simulink model "FitzHugh_Nagumo"  (R2014b)
settings: Solver=ode45  StartTime=0.0  StopTime=100.0  RelTol=1e-3
values from neighbouring files (symbols this model uses):
  a = 0.95    [Run_Aizawa.m]    (also in Run_Arneodo.m = -5.5; Run_Chen.m = 33; Run_Chua.m = 15.6; Run_Chua_4D.m = 0.03)
  A = 30    [Run_Chua_4D.m]    (also in Run_FitzHugh_Nagumo.m = 0.8)
  b = 0.7    [Run_Aizawa.m]    (also in Run_Arneodo.m = 3.5; Run_Chen.m = 3; Run_Chua.m = 28; Run_Duffing.m = 100)
  e = 0.15    [Run_Aizawa.m]    (also in Run_Belousov_Zhabotinsky.m = 0.3; Run_Dadras.m = 9; Run_FitzHugh_Nagumo.m = 0.1)
  omega = 0.7    [Run_FitzHugh_Nagumo.m]
undefined symbols (not defined in the file or in its folder): param
settings Model: Creator=Arek  LastModifiedBy=Arek

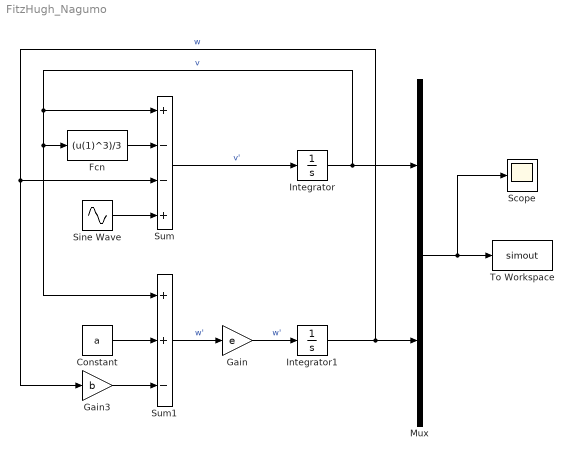
== system FitzHugh_Nagumo ==
  Constant : Constant  Value=a
  Fcn : Fcn  Expr=(u(1)^3)/3
  Gain : Gain  Gain=e
  Gain3 : Gain  Gain=b
  Integrator : Integrator  InitialCondition=param.ic(1)
  Integrator1 : Integrator  InitialCondition=param.ic(2)
  Mux : Mux  Inputs=2
  Scope : Scope
      settings: ShowLegends=on
  Sine Wave : Sin  Amplitude=A  Frequency=omega  SampleTime=0
  Sum : Sum  Inputs=+--+
  Sum1 : Sum  Inputs=++-
  To Workspace : ToWorkspace  VariableName=simout  SaveFormat=Timeseries  SampleTime=-1
  wires:
  Integrator/1 -> Sum/1, Fcn/1, Sum1/1, Mux/1  "v"
  Gain/1 -> Integrator1/1  "w'"
  Integrator1/1 -> Mux/2, Sum/3, Gain3/1  "w"
  Mux/1 -> To Workspace/1, Scope/1
  Sum/1 -> Integrator/1  "v'"
  Fcn/1 -> Sum/2
  Sine Wave/1 -> Sum/4
  Sum1/1 -> Gain/1  "w'"
  Constant/1 -> Sum1/2
  Gain3/1 -> Sum1/3
